simulink model "simF16"  (R2014a)
settings: Solver=ode45  StartTime=0.0  StopTime=10.0  RelTol=1e-3
values from neighbouring files (symbols this model uses):
  A = f16ss.a    [h2F16.m]    (also in h2F16ex2.m; h2F16ex3.m; h2F16ex_iconnect.m; h2cart.m = [0 0 1 0)
  B = [Bd Bu]    [h2F16.m]    (also in h2F16ex2.m = [Bu Bd]; h2F16ex3.m; h2F16ex_iconnect.m; hinfF16.m = [Bu Bd])
  h2K = Z*inv(X)    [h2F16.m]    (also in h2F16ex2.m; h2F16ex3.m; h2cart.m; h2ex1.m)
  nd = 1    [h2F16.m]    (also in h2F16ex2.m; h2F16ex3.m; h2F16ex_iconnect.m)
  nu = 2    [h2F16.m]    (also in h2F16ex2.m; h2F16ex3.m; h2F16ex_iconnect.m; h2cart.m = 1)
  nx = 4    [h2F16.m]    (also in h2F16ex2.m; h2F16ex3.m; h2F16ex_iconnect.m; h2cart.m)
settings Model: Creator=raktim  LastModifiedBy=raktim

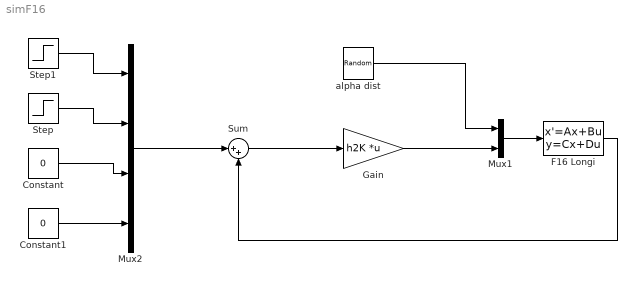
== system simF16 ==
  Constant : Constant  Value=0
  Constant1 : Constant  Value=0
  F16 Longi : StateSpace  A=A  B=B  C=eye(nx)  D=zeros(nx,nd+nu)  X0=0
  Gain : Gain  Gain=h2K  Multiplication=Matrix(K*u)
  Mux1 : Mux  Inputs=2
  Mux2 : Mux
  Step : Step  SampleTime=0
  Step1 : Step  SampleTime=0
  Sum : Sum  Inputs=|++
  alpha dist : UniformRandomNumber  SampleTime=0.1
  wires:
  F16 Longi/1 -> Sum/2
  Sum/1 -> Gain/1
  Mux1/1 -> F16 Longi/1
  alpha dist/1 -> Mux1/1
  Gain/1 -> Mux1/2
  Constant1/1 -> Mux2/4
  Constant/1 -> Mux2/3
  Step/1 -> Mux2/2
  Step1/1 -> Mux2/1
  Mux2/1 -> Sum/1
